simulink model "speed_regulator_ROCOF_r2022a"  (R2022a)
settings: Solver=ode4  StartTime=0.0  StopTime=Inf  FixedStep=0.4  RelTol=1e-3  AbsTol=1e-6
undefined symbols (not defined in the file): Continuous, Efd0, Efd1, Efd2, gcbh, Ka, Ke, Kf, SeEfd1, SeEfd2, sps_rtmsupport, spsAC5AModel, Ta, Te, Tf1, Tf2, Tf3, VR0, VRmax, VRmin
libraries: simulink x1, simulink_extras x1
settings Model: Creator=dmedonza  LastModifiedBy=stefanocassano
settings SolverCC: AutoScaleAbsTol=off  AlgebraicLoopSolver=TrustRegion
settings DataIOCC: LimitDataPoints=on  SaveFormat=Array  SignalLoggingSaveFormat=ModelDataLogs  SaveOutput=off  SignalLogging=off  SaveTime=off  ReturnWorkspaceOutputs=off
settings OptimizationCC: BooleanDataType=off  ExpressionDepthLimit=2147483647  LifeSpan=inf
settings DebuggingCC: SaveWithParameterizedLinksMsg=none  UnderspecifiedInitializationDetection=Classic  MergeDetectMultiDrivingBlocksExec=none  SignalResolutionControl=TryResolveAllWithWarning  MultiTaskDSMMsg=warning  MultiTaskCondExecSysMsg=none  FcnCallInpInsideContextMsg=warning  UnconnectedInputMsg=warning  UnconnectedOutputMsg=warning  UnconnectedLineMsg=warning  StateNameClashWarn=warning  SFUnexpectedBacktrackingDiag=warning  SFNoUnconditionalDefaultTransitionDiag=warning  SFExecutionAtInitializationDiag=none  ArithmeticOperatorsInVariantConditions=warning
settings HardwareCC: ProdBitPerPointer=32  ProdBitPerSizeT=32  ProdBitPerPtrDiffT=32  ProdLargestAtomicFloat=None  ProdIntDivRoundTo=Undefined  ProdEndianess=Unspecified  ProdWordSize=32  ProdHWDeviceType=32-bit Generic  TargetUnknown=on
settings ModelReferenceCC: EnableRefExpFcnMdlSchedulingChecks=off  PropagateSignalLabelsOutOfModel=off
settings SFSimCC: SimUseLocalCustomCode=off  CustomCodeUndefinedFunction=UseInterfaceOnly
settings RTWCC: TemplateMakefile=grt_vc.tmf  RTWUseLocalCustomCode=off
settings CodeAppCC: StateflowObjectComments=on
settings GRTTargetCC: TargetLangStandard=C89/C90 (ANSI)  CombineOutputUpdateFcns=off  GRTInterface=on
settings ConfigComp: CovMetricSettings=dw  CovSaveCumulativeToWorkspaceVar=on  CovSaveSingleToWorkspaceVar=on  CovExternalEMLEnable=off

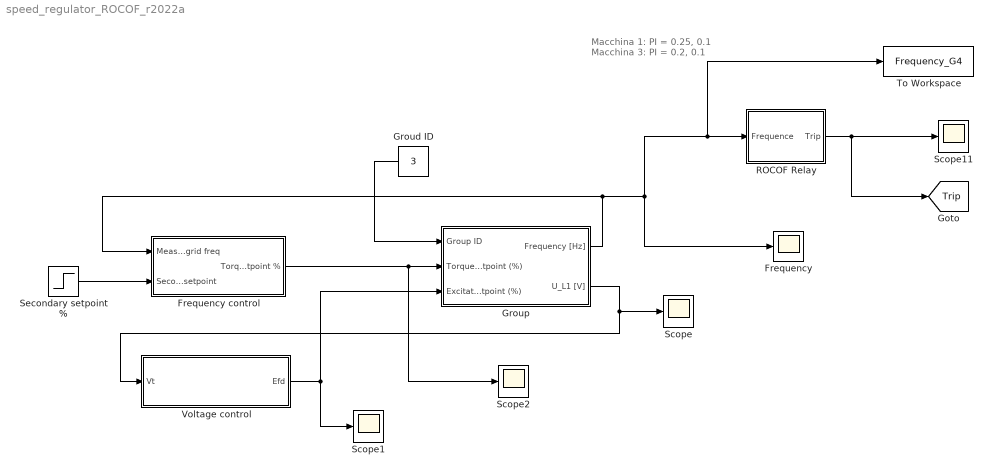
== system speed_regulator_ROCOF_r2022a ==
  note: Macchina 1: PI = 0.25, 0.1
      | Macchina 3: PI = 0.2, 0.1
  Frequency : Scope
  Frequency control : Subsystem
  Groud ID : Constant  Value=3
  Group : Subsystem
  ROCOF Relay : Subsystem
  Scope{,1..2,11} (4 alike) : Scope
  Secondary setpoint % : Step  Time=550  Before=0.04  After=0.10  SampleTime=0
  To Workspace : ToWorkspace  VariableName=Frequency_G4  SaveFormat=Timeseries  SampleTime=-1
  Voltage control : Subsystem
  tag scope: Trip=global
  wires:
  Groud ID/1 -> Group/1(Group ID)
  Group/2(U_L1 [V]) -> Voltage control/1(Vt), Scope/1
  Voltage control/1(Efd) -> Group/3(Excitation setpoint (%)), Scope1/1
  Secondary setpoint %/1 -> Frequency control/2(Secondary setpoint)
  Group/1(Frequency [Hz]) -> Frequency control/1(Measured grid freq), Frequency/1, To Workspace/1, ROCOF Relay/1(Frequence)
  Frequency control/1("Torque setpoint % ") -> Scope2/1, Group/2(Torque setpoint (%))
  ROCOF Relay/1(Trip) -> [Trip], Scope11/1

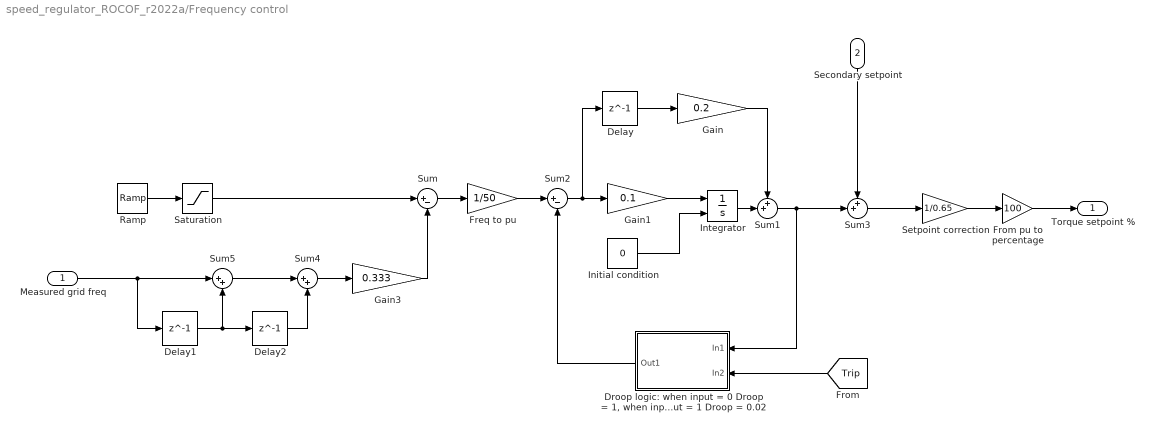
== system speed_regulator_ROCOF_r2022a/Frequency control ==
  Measured grid freq : Inport
  Secondary setpoint : Inport  Port=2
  " Setpoint correction " : Gain  Gain=1/0.65
  Delay : Delay  DelayLength=1  InitialCondition=0
  Delay1 : Delay  DelayLength=1  InitialCondition=0
  Delay2 : Delay  DelayLength=1  InitialCondition=0
  "Droop logic: when input = 0 Droop = 1, when input = 1 Droop = 0.02" : Subsystem
  Freq to pu : Gain  Gain=1/50
  From pu to percentage : Gain  Gain=100
  Gain : Gain  Gain=0.2
  Gain1 : Gain  Gain=0.1
  Gain3 : Gain  Gain=0.333
  Initial condition : Constant  Value=0
  Integrator : Integrator  InitialConditionSource=external
  Ramp : simulink/Sources/Ramp  slope=2  start=0  InitialOutput=0
  Saturation : Saturate  UpperLimit=50  LowerLimit=0
  Sum : Sum  Inputs=|+-
  Sum1 : Sum  Inputs=++|
  Sum2 : Sum  Inputs=|+-
  Sum3 : Sum  Inputs=++|
  Sum4 : Sum  Inputs=|++
  Sum5 : Sum  Inputs=|++
  "Torque setpoint % " : Outport
  wires:
  Initial condition/1 -> Integrator/2
  Delay/1 -> Gain/1
  Ramp/1 -> Saturation/1
  Sum2/1 -> Delay/1, Gain1/1
  Gain1/1 -> Integrator/1
  Gain/1 -> Sum1/1
  Integrator/1 -> Sum1/2
  Measured grid freq/1 -> Sum5/1, Delay1/1
  Gain3/1 -> Sum/2
  Delay1/1 -> Delay2/1, Sum5/2
  Sum/1 -> Freq to pu/1
  Sum5/1 -> Sum4/1
  Delay2/1 -> Sum4/2
  Sum4/1 -> Gain3/1
  Secondary setpoint/1 -> Sum3/1
  "Droop logic: when input = 0 Droop = 1, when input = 1 Droop = 0.02"/1(Out1) -> Sum2/2
  Freq to pu/1 -> Sum2/1
  Sum1/1 -> Sum3/2, "Droop logic: when input = 0 Droop = 1, when input = 1 Droop = 0.02"/1(In1)
  Sum3/1 -> " Setpoint correction "/1
  [Trip] -> "Droop logic: when input = 0 Droop = 1, when input = 1 Droop = 0.02"/2(In2)
  " Setpoint correction "/1 -> From pu to percentage/1
  From pu to percentage/1 -> "Torque setpoint % "/1
  Saturation/1 -> Sum/1

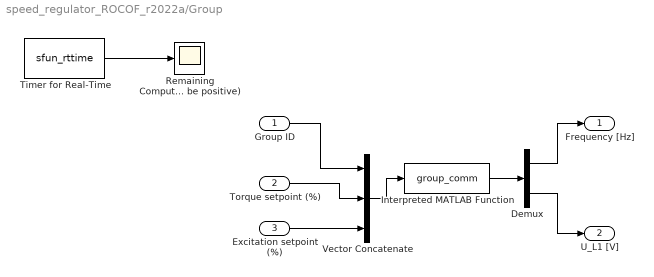
== system speed_regulator_ROCOF_r2022a/Group ==
  Group ID : Inport
  Torque setpoint (%) : Inport  Port=2
  Excitation setpoint (%) : Inport  Port=3
  Demux : Demux  Outputs=2
  Interpreted MATLAB Function : MATLABFcn  MATLABFcn=group_comm  OutputDimensions=2
  Remaining Computation Time (must be positive) : Scope
  Timer for Real-Time : S-Function  FunctionName=sfun_rttime  Parameters=1  SFunctionDeploymentMode=off  EnableBusSupport=off
  Vector Concatenate : Concatenate  NumInputs=3
  Frequency [Hz] : Outport
  U_L1 [V] : Outport  Port=2
  wires:
  Torque setpoint (%)/1 -> Vector Concatenate/2
  Group ID/1 -> Vector Concatenate/1
  Vector Concatenate/1 -> Interpreted MATLAB Function/1
  Interpreted MATLAB Function/1 -> Demux/1
  Timer for Real-Time/1 -> Remaining Computation Time (must be positive)/1
  Demux/1 -> Frequency [Hz]/1
  Excitation setpoint (%)/1 -> Vector Concatenate/3
  Demux/2 -> U_L1 [V]/1

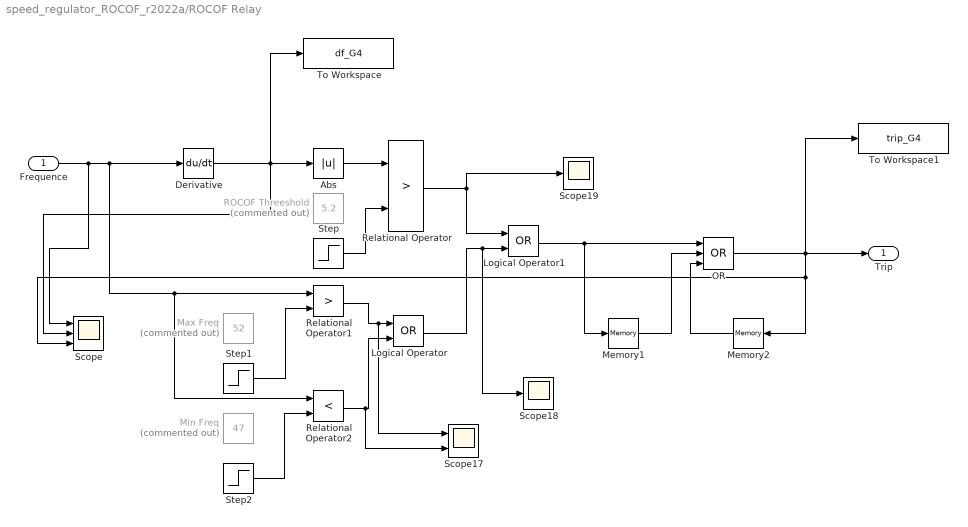
== system speed_regulator_ROCOF_r2022a/ROCOF Relay ==
  Frequence : Inport
  Abs : Abs  SaturateOnIntegerOverflow=off
  Derivative : Derivative
  Logical Operator : Logic  Operator=OR  AllPortsSameDT=off  OutDataTypeStr=boolean
  Logical Operator1 : Logic  Operator=OR  AllPortsSameDT=off  OutDataTypeStr=boolean
  Max Freq : Constant  Commented=on  Value=52
  Memory1 : Memory
  Memory2 : Memory
  Min Freq : Constant  Commented=on  Value=47
  OR : Logic  Operator=OR  Inputs=3  IconShape=distinctive  AllPortsSameDT=off  OutDataTypeStr=boolean
  ROCOF Threeshold : Constant  Commented=on  Value=5.2
  Relational Operator : RelationalOperator  Operator=>  OutDataTypeStr=boolean  RndMeth=Simplest  InputSameDT=off
  Relational Operator1 : RelationalOperator  Operator=>  OutDataTypeStr=boolean  RndMeth=Simplest  InputSameDT=off
  Relational Operator2 : RelationalOperator  Operator=<  OutDataTypeStr=boolean  RndMeth=Simplest  InputSameDT=off
  Scope : Scope  NumInputPorts=3
  Scope17 : Scope  NumInputPorts=2
  Scope18 : Scope
  Scope19 : Scope
  Step : Step  Time=50  Before=5.5e5  After=2.8  SampleTime=0
  Step1 : Step  Time=50  Before=600  After=52  SampleTime=0
  Step2 : Step  Time=50  Before=-600  After=47  SampleTime=0
  To Workspace : ToWorkspace  VariableName=df_G4  SaveFormat=Timeseries  SampleTime=-1
  To Workspace1 : ToWorkspace  VariableName=trip_G4  SaveFormat=Timeseries  SampleTime=-1
  Trip : Outport
  wires:
  Frequence/1 -> Scope/1, Derivative/1, Relational Operator1/1, Relational Operator2/1
  Logical Operator/1 -> Scope18/1, Logical Operator1/2
  Relational Operator1/1 -> Scope17/1, Logical Operator/1
  Relational Operator2/1 -> Scope17/2, Logical Operator/2
  Relational Operator/1 -> Logical Operator1/1, Scope19/1
  Abs/1 -> Relational Operator/1
  Derivative/1 -> To Workspace/1, Scope/2, Abs/1
  OR/1 -> Scope/3, Memory2/1, To Workspace1/1, Trip/1
  Memory1/1 -> OR/2
  Logical Operator1/1 -> OR/1, Memory1/1
  Memory2/1 -> OR/3
  Step/1 -> Relational Operator/2
  Step2/1 -> Relational Operator2/2
  Step1/1 -> Relational Operator1/2

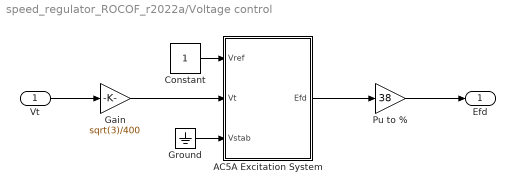
== system speed_regulator_ROCOF_r2022a/Voltage control ==
  Vt : Inport
  AC5A Excitation System : Subsystem  AncestorBlock=sps_lib/Electrical Machines/Synchronous Machine Control/AC5A Excitation System  DialogController=POWERSYS.PowerSysDialog  LoadFcn=sps_rtmsupport('LoadFcn', gcbh);  StartFcn=sps_rtmsupport('StartFcn', gcbh);  StopFcn=sps_rtmsupport('StopFcn', gcbh);  mask(AC5A Excitation System){Tr=20e-4, KaTa=[1 0.2], VRminmax=[-5.3 5.3], KfTf=[0.3 1 0 0], KeTe=[1.0 0.25], Efd12=[7 0.75*7], SeEfd12=[0.86 0.5], v0=[1 1], TsBlock=0}
      mask prompts: Tr "Low-pass filter time constant Tr(s):"; KaTa "Voltage regulator gain and time constant [Ka Ta(s)]:"; VRminmax "Voltage regulator output limits [VRmin(pu) VRmax(pu)]:"; KfTf "Damping filter gain and time constants [Kf Tf1(s) Tf2(s) Tf3(s)]:"; KeTe "Exciter gain and time constant [Ke Te(s)]:"; Efd12 "Field voltage values [Efd1(pu) Efd2(pu)]:"; SeEfd12 "Exciter saturation function values [SeEfd1(pu) SeEfd2(pu)]:"; v0 "Initial values of terminal voltage and field voltage [Vt0(pu) Efd0(pu)]:"; TsBlock "Sample time:"
      mask help: Implements a synchronous machine voltage regulator and exciter based on the IEEE type AC5A excitation system model. The output is the field voltage to apply to the Vf input of a Synchronous Machine block. Inputs and output are in p.u.
      mask init:
      | block = gcb;
      | [Ts,BlockChoice,MaskType,Ka,Ta,Ke,Te,Kf,Tf1,Tf2,Tf3,Efd1,Efd2,SeEfd1,SeEfd2,VRmin,VRmax,Vt0,Efd0,VR0] = powericon('ExcitationSystemInit',block,TsBlock,KaTa,KeTe,KfTf,Efd12,SeEfd12,VRminmax,v0);
      | powericon('SetInternalModels','set',block,BlockChoice);
      settings: CopyFcn=sps_rtmsupport('CopyFcn', gcbh);  DeleteFcn=sps_rtmsupport('DeleteFcn', gcbh);  UndoDeleteFcn=sps_rtmsupport('UndoDeleteFcn', gcbh);  ModelCloseFcn=sps_rtmsupport('ModelCloseFcn', gcbh);  PreSaveFcn=sps_rtmsupport('PreSaveFcn', gcbh);  PostSaveFcn=sps_rtmsupport('PostSaveFcn', gcbh);  NameChangeFcn=sps_rtmsupport('NameChangeFcn', gcbh);  PreCopyFcn=sps_rtmsupport('PreCopyFcn', gcbh);  OpenFcn=sps_rtmsupport('OpenFcn', gcbh, []);  CloseFcn=sps_rtmsupport('CloseFcn', gcbh);  PreDeleteFcn=sps_rtmsupport('PreDeleteFcn', gcbh);
      mask Help: helpview(psbhelp);
      mask Display: color('blue');disp('AC5A')
  Constant : Constant
  Gain : Gain  Gain=sqrt(3)/400
  Ground : Ground
  Pu to % : Gain  Gain=38
  Efd : Outport
  wires:
  Ground/1 -> AC5A Excitation System/3(Vstab)
  Vt/1 -> Gain/1
  AC5A Excitation System/1(Efd) -> Pu to %/1
  Constant/1 -> AC5A Excitation System/1(Vref)
  Pu to %/1 -> Efd/1
  Gain/1 -> AC5A Excitation System/2(Vt)

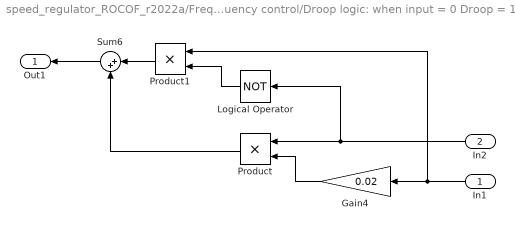
== system speed_regulator_ROCOF_r2022a/Frequency control/Droop logic: when input = 0 Droop = 1, when input = 1 Droop = 0.02 ==
  In1 : Inport
  In2 : Inport  Port=2
  Gain4 : Gain  Gain=0.02
  Logical Operator : Logic  Operator=NOT  AllPortsSameDT=off  OutDataTypeStr=boolean
  Product : Product
  Product1 : Product
  Sum6 : Sum  Inputs=|++
  Out1 : Outport
  wires:
  Sum6/1 -> Out1/1
  Gain4/1 -> Product/2
  In1/1 -> Product1/1, Gain4/1
  Product/1 -> Sum6/2
  In2/1 -> Logical Operator/1, Product/1
  Logical Operator/1 -> Product1/2
  Product1/1 -> Sum6/1

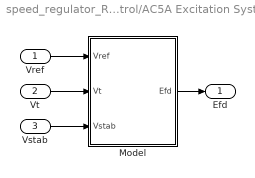
== system speed_regulator_ROCOF_r2022a/Voltage control/AC5A Excitation System ==
  Vref : Inport
  Vt : Inport  Port=2
  Vstab : Inport  Port=3
  Model : Subsystem  AncestorBlock=spsAC5AModel/Continuous  mask(Excitation System){}
  Efd : Outport  VectorParamsAs1DForOutWhenUnconnected=off
  wires:
  Model/1(Efd) -> Efd/1
  Vref/1 -> Model/1(Vref)
  Vt/1 -> Model/2(Vt)
  Vstab/1 -> Model/3(Vstab)

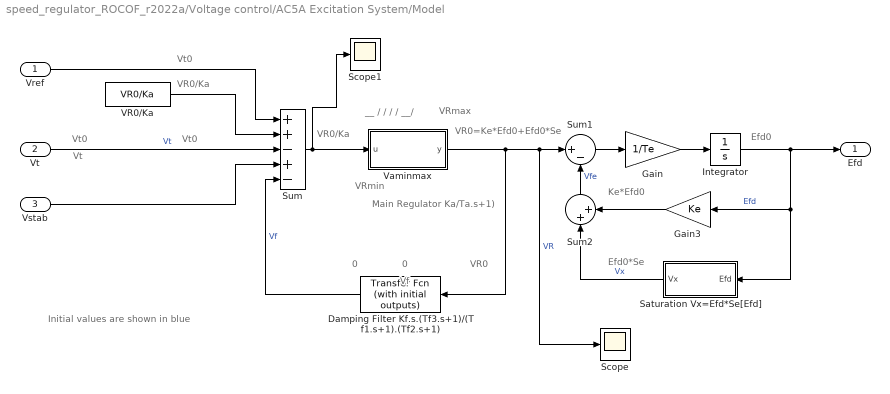
== system speed_regulator_ROCOF_r2022a/Voltage control/AC5A Excitation System/Model ==
  note: VRmax
  note: VRmin
  note: __
      |              /
      |           /
      |         /
      |       /
      | __/
  note: Main Regulator
      | Ka/Ta.s+1)
  note: VR0/Ka
  note: Efd0
  note: Ke*Efd0
  note: Efd0*Se
  note: VR0
  note: 0
  note: VR0=Ke*Efd0+Efd0*Se
  note: Vt0
  note: Vt0
  note: VR0/Ka
  note: Initial values are shown in blue
  note: Vf
  note: 0
  note: Vt0
  note: Vt
  Vref : Inport
  Vt : Inport  Port=2
  Vstab : Inport  Port=3
  Damping Filter Kf.s.(Tf3.s+1)/(Tf1.s+1).(Tf2.s+1) : simulink_extras/Additional Linear/Transfer Fcn (with initial outputs)  N=[Kf*Tf3 Kf 0]  D=[Tf1*Tf2 (Tf1+Tf2) 1]  Y0=0  U0=VR0
  Gain : Gain  Gain=1/Te  SaturateOnIntegerOverflow=on  OutDataTypeStr=Inherit: Same as input  ParamDataTypeStr=Inherit: Same as input
  Gain3 : Gain  Gain=Ke  SaturateOnIntegerOverflow=on  OutDataTypeStr=Inherit: Same as input  ParamDataTypeStr=Inherit: Same as input
  Integrator : Integrator  InitialCondition=Efd0  LimitOutput=on  LowerSaturationLimit=0
  Saturation Vx=Efd*Se[Efd] : Subsystem  mask{Efd12=[Efd1 Efd2], SeEfd12=[SeEfd1 SeEfd2]}
      mask prompts: Efd12 "Field voltage values [Efd1(pu) Efd2(pu)]:"; SeEfd12 "Exciter saturation function values [SeEfd1(pu) SeEfd2(pu)]:"
      mask init:
      | Efd1 = Efd12(1);Efd2 = Efd12(2);
      | SeEfd1 = SeEfd12(1);SeEfd2 = SeEfd12(2);
  Scope : Scope
  Scope1 : Scope
  Sum : Sum  Inputs=++-+-  InputSameDT=on  SaturateOnIntegerOverflow=on  OutDataTypeStr=Inherit: Same as first input
  Sum1 : Sum  Inputs=|+-
  Sum2 : Sum  Inputs=|++
  VR0/Ka : Constant  Value=VR0/Ka
  Vaminmax : Subsystem  mask{Ka=Ka, Ta=Ta, VRminmax=[VRmin VRmax], X0=VR0}
      mask prompts: Ka "Voltage regulator gain Ka:"; Ta "Voltage regulator time constant Ta(s):"; VRminmax "Voltage regulator output limits [VRmin(pu) VRmax(pu)]:"; X0 "Initial conditions:"
      mask init:
      | VRmin=VRminmax(1);VRmax=VRminmax(2);
      mask Display: dpoly([Ka],[Ta 1],'s')
  Efd : Outport  VectorParamsAs1DForOutWhenUnconnected=off
  wires:
  Gain/1 -> Integrator/1
  Saturation Vx=Efd*Se[Efd]/1(Vx) -> Sum2/1  "Vx"
  Gain3/1 -> Sum2/2
  Integrator/1 -> Efd/1, Saturation Vx=Efd*Se[Efd]/1(Efd), Gain3/1  "Efd"
  Sum2/1 -> Sum1/2  "Vfe"
  Sum1/1 -> Gain/1
  Sum/1 -> Scope1/1, Vaminmax/1(u)
  Vaminmax/1(y) -> Damping Filter Kf.s.(Tf3.s+1)/(Tf1.s+1).(Tf2.s+1)/1, Scope/1, Sum1/1  "VR"
  Vref/1 -> Sum/1
  VR0/Ka/1 -> Sum/2
  Vt/1 -> Sum/3  "Vt"
  Vstab/1 -> Sum/4
  Damping Filter Kf.s.(Tf3.s+1)/(Tf1.s+1).(Tf2.s+1)/1 -> Sum/5  "Vf"

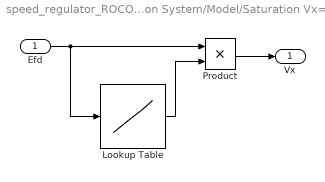
== system speed_regulator_ROCOF_r2022a/Voltage control/AC5A Excitation System/Model/Saturation Vx=Efd*Se[Efd] ==
  Efd : Inport
  Lookup Table : Lookup_n-D  NumberOfTableDimensions=1  BreakpointsForDimension1=[0 Efd2 Efd1]  Table=[0 SeEfd2 SeEfd1]  InternalRulePriority=Speed  RndMeth=Simplest
  Product : Product  RndMeth=Zero
  Vx : Outport  VectorParamsAs1DForOutWhenUnconnected=off
  wires:
  Lookup Table/1 -> Product/2
  Product/1 -> Vx/1
  Efd/1 -> Product/1, Lookup Table/1

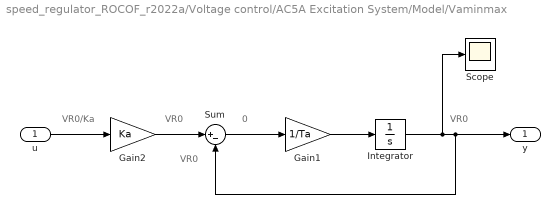
== system speed_regulator_ROCOF_r2022a/Voltage control/AC5A Excitation System/Model/Vaminmax ==
  note: VR0
  note: 0
  note: VR0
  note: VR0
  note: VR0/Ka
  u : Inport
  Gain1 : Gain  Gain=1/Ta  SaturateOnIntegerOverflow=on  OutDataTypeStr=Inherit: Same as input  ParamDataTypeStr=Inherit: Same as input
  Gain2 : Gain  Gain=Ka  SaturateOnIntegerOverflow=on  OutDataTypeStr=Inherit: Same as input  ParamDataTypeStr=Inherit: Same as input
  Integrator : Integrator  InitialCondition=VR0  LimitOutput=on  UpperSaturationLimit=VRmax  LowerSaturationLimit=VRmin
  Scope : Scope
  Sum : Sum  Inputs=|+-  InputSameDT=on  SaturateOnIntegerOverflow=on  OutDataTypeStr=Inherit: Same as first input
  y : Outport  VectorParamsAs1DForOutWhenUnconnected=off
  wires:
  Gain1/1 -> Integrator/1
  Gain2/1 -> Sum/1
  Integrator/1 -> Scope/1, Sum/2, y/1
  Sum/1 -> Gain1/1
  u/1 -> Gain2/1
